simulink model "force_interaction"  (R2016b)
settings: Solver=FixedStepDiscrete  StartTime=0.0  StopTime=10  FixedStep=0.002  RelTol=1e-3
values from neighbouring files (symbols this model uses):
  r_kd = 1.0    [force_interaction.sldd]    (also in init.m = 0)
  r_ki = 1.0    [force_interaction.sldd]    (also in init.m = 0)
  r_kp = 1.0    [force_interaction.sldd]    (also in init.m = 0)
  x_kd = 1.0    [force_interaction.sldd]    (also in init.m = 0)
  x_ki = 1.0    [force_interaction.sldd]    (also in init.m = 0)
  x_kp = 1.0    [force_interaction.sldd]    (also in init.m = 100)
  x_rate = 1000/250    (= 4)    [init.m]
libraries: cstblocks x6, simulink x4
settings Model: Creator=gaoxiao  LastModifiedBy=gx
settings OptimizationCC: DefaultParameterBehavior=Inlined  ZeroExternalMemoryAtStartup=off
settings DebuggingCC: ParameterTunabilityLossMsg=error
settings RTWCC: SystemTargetFile=ert.tlc  GenCodeOnly=on  GenerateMakefile=off  TemplateMakefile=RTW.MSVCBuild  Description=Create Visual C/C++ Solution File for Embedded Coder  GenerateReport=on  IncludeHyperlinkInReport=on  LaunchReport=on  TargetLang=C++  GenerateTraceInfo=on  GenerateTraceReport=on  GenerateTraceReportSl=on  GenerateTraceReportSf=on  GenerateTraceReportEml=on  GenerateWebview=on  GenerateCodeMetricsReport=on
settings CodeAppCC: ForceParamTrailComments=on  OperatorAnnotations=on  SimulinkDataObjDesc=on  SFDataObjDesc=on  MATLABFcnDesc=on  InsertBlockDesc=on  MATLABSourceComments=on
settings ERTTargetCC: TargetLangStandard=C++03 (ISO)  GenerateSampleERTMain=on  MultiInstanceERTCode=on  CodeInterfacePackaging=C++ class  InlinedParameterPlacement=NonHierarchical  RootIOFormat=Structure reference  ERTCustomFileTemplate=example_file_process.tlc  ERTFilePackagingFormat=Compact

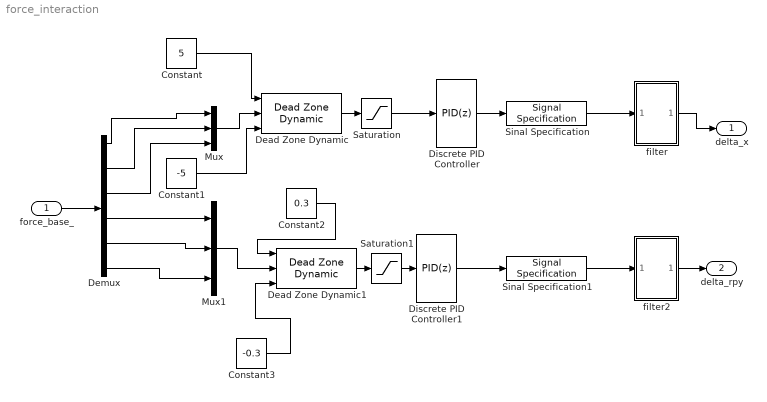
== system force_interaction ==
  force_base_ : Inport  PortDimensions=6
  Constant : Constant  Value=5
  Constant1 : Constant  Value=-5
  Constant2 : Constant  Value=0.3
  Constant3 : Constant  Value=-0.3
  Dead Zone Dynamic : simulink/Discontinuities/Dead Zone Dynamic
  Dead Zone Dynamic1 : simulink/Discontinuities/Dead Zone Dynamic
  Demux : Demux  Outputs=6
  Discrete PID Controller : simulink/Continuous/PID Controller  Controller=PID  TimeDomain=Discrete-time  SampleTime=-1  IntegratorMethod=Forward Euler  FilterMethod=Forward Euler  Form=Parallel  UseFilter=on  ControllerParametersSource=internal  P=x_kp  I=x_ki  D=x_kd  N=5  InitialConditionSource=internal  InitialConditionForIntegrator=0  InitialConditionForFilter=0  ExternalReset=none  LimitOutput=off  UpperSaturationLimit=inf  LowerSaturationLimit=-inf  LinearizeAsGain=off  AntiWindupMode=none  Kb=1  TrackingMode=off  Kt=1  PParamMin=[]  PParamMax=[]  IParamMin=[]  IParamMax=[]  DParamMin=[]  DParamMax=[]  NParamMin=[]  NParamMax=[]  KbParamMin=[]  KbParamMax=[]  KtParamMin=[]  KtParamMax=[]  POutMin=[]  POutMax=[]  IOutMin=[]  IOutMax=[]  DOutMin=[]  DOutMax=[]  NOutMin=[]  NOutMax=[]  KbOutMin=[]  KbOutMax=[]  KtOutMin=[]  KtOutMax=[]  IntegratorOutMin=[]  IntegratorOutMax=[]  FilterOutMin=[]  FilterOutMax=[]  SumOutMin=[]  SumOutMax=[]  SumI1OutMin=[]  SumI1OutMax=[]  SumI2OutMin=[]  SumI2OutMax=[]  SumI3OutMin=[]  SumI3OutMax=[]  SumDOutMin=[]  SumDOutMax=[]  SaturationOutMin=[]  SaturationOutMax=[]  IntegratorContinuousStateAttributes=''  IntegratorStateMustResolveToSignalObject=off  IntegratorRTWStateStorageClass=Auto  FilterContinuousStateAttributes=''  FilterStateMustResolveToSignalObject=off  FilterRTWStateStorageClass=Auto  DifferentiatorICPrevScaledInput=0  DifferentiatorOutMin=[]  DifferentiatorOutMax=[]
  Discrete PID Controller1 : simulink/Continuous/PID Controller  Controller=PID  TimeDomain=Discrete-time  SampleTime=-1  IntegratorMethod=Forward Euler  FilterMethod=Forward Euler  Form=Parallel  UseFilter=on  ControllerParametersSource=internal  P=r_kp  I=r_ki  D=r_kd  N=5  InitialConditionSource=internal  InitialConditionForIntegrator=0  InitialConditionForFilter=0  ExternalReset=none  LimitOutput=off  UpperSaturationLimit=inf  LowerSaturationLimit=-inf  LinearizeAsGain=off  AntiWindupMode=none  Kb=1  TrackingMode=off  Kt=1  PParamMin=[]  PParamMax=[]  IParamMin=[]  IParamMax=[]  DParamMin=[]  DParamMax=[]  NParamMin=[]  NParamMax=[]  KbParamMin=[]  KbParamMax=[]  KtParamMin=[]  KtParamMax=[]  POutMin=[]  POutMax=[]  IOutMin=[]  IOutMax=[]  DOutMin=[]  DOutMax=[]  NOutMin=[]  NOutMax=[]  KbOutMin=[]  KbOutMax=[]  KtOutMin=[]  KtOutMax=[]  IntegratorOutMin=[]  IntegratorOutMax=[]  FilterOutMin=[]  FilterOutMax=[]  SumOutMin=[]  SumOutMax=[]  SumI1OutMin=[]  SumI1OutMax=[]  SumI2OutMin=[]  SumI2OutMax=[]  SumI3OutMin=[]  SumI3OutMax=[]  SumDOutMin=[]  SumDOutMax=[]  SaturationOutMin=[]  SaturationOutMax=[]  IntegratorContinuousStateAttributes=''  IntegratorStateMustResolveToSignalObject=off  IntegratorRTWStateStorageClass=Auto  FilterContinuousStateAttributes=''  FilterStateMustResolveToSignalObject=off  FilterRTWStateStorageClass=Auto  DifferentiatorICPrevScaledInput=0  DifferentiatorOutMin=[]  DifferentiatorOutMax=[]
  Mux : Mux  Inputs=3
  Mux1 : Mux  Inputs=3
  Saturation : Saturate  UpperLimit=40  LowerLimit=-40
  Saturation1 : Saturate  UpperLimit=3  LowerLimit=-3
  Sinal Specification : SignalSpecification  OutDataTypeStr=double  Dimensions=3
  Sinal Specification1 : SignalSpecification  OutDataTypeStr=double  Dimensions=3
  filter : Subsystem
  filter2 : Subsystem
  delta_x : Outport  PortDimensions=3
  delta_rpy : Outport  Port=2  PortDimensions=3
  wires:
  Discrete PID Controller/1 -> Sinal Specification/1
  force_base_/1 -> Demux/1
  Demux/5 -> Mux1/2
  Demux/4 -> Mux1/1
  Demux/6 -> Mux1/3
  Demux/1 -> Mux/1
  Demux/2 -> Mux/2
  Demux/3 -> Mux/3
  Mux/1 -> Dead Zone Dynamic/2
  Discrete PID Controller1/1 -> Sinal Specification1/1
  Mux1/1 -> Dead Zone Dynamic1/2
  Constant/1 -> Dead Zone Dynamic/1
  Constant1/1 -> Dead Zone Dynamic/3
  Constant2/1 -> Dead Zone Dynamic1/1
  Constant3/1 -> Dead Zone Dynamic1/3
  Dead Zone Dynamic/1 -> Saturation/1
  Saturation/1 -> Discrete PID Controller/1
  Dead Zone Dynamic1/1 -> Saturation1/1
  Saturation1/1 -> Discrete PID Controller1/1
  Sinal Specification/1 -> filter/1(In1)
  filter/1(Out1) -> delta_x/1
  Sinal Specification1/1 -> filter2/1(In1)
  filter2/1(Out1) -> delta_rpy/1

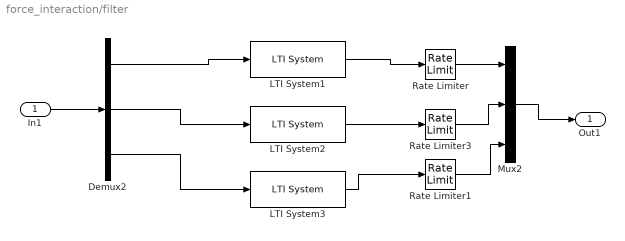
== system force_interaction/filter ==
  In1 : Inport
  Demux2 : Demux  Outputs=3
  LTI System1 : cstblocks/LTI System  sys=TT  IC=[]
  LTI System2 : cstblocks/LTI System  sys=TT  IC=[]
  LTI System3 : cstblocks/LTI System  sys=TT  IC=[]
  Mux2 : Mux  Inputs=3
  Rate Limiter : RateLimiter  RisingSlewLimit=x_rate  FallingSlewLimit=-x_rate  SampleTimeMode=inherited
  Rate Limiter1 : RateLimiter  RisingSlewLimit=x_rate  FallingSlewLimit=-x_rate  SampleTimeMode=inherited
  Rate Limiter3 : RateLimiter  RisingSlewLimit=x_rate  FallingSlewLimit=-x_rate  SampleTimeMode=inherited
  Out1 : Outport
  wires:
  Demux2/2 -> LTI System2/1
  Demux2/1 -> LTI System1/1
  Demux2/3 -> LTI System3/1
  Mux2/1 -> Out1/1
  Rate Limiter3/1 -> Mux2/2
  LTI System3/1 -> Rate Limiter1/1
  Rate Limiter1/1 -> Mux2/3
  Rate Limiter/1 -> Mux2/1
  LTI System2/1 -> Rate Limiter3/1
  LTI System1/1 -> Rate Limiter/1
  In1/1 -> Demux2/1

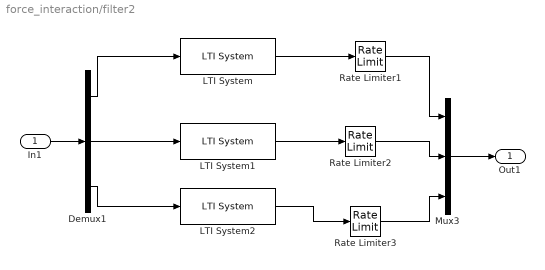
== system force_interaction/filter2 ==
  In1 : Inport
  Demux1 : Demux  Outputs=3
  LTI System : cstblocks/LTI System  sys=TT  IC=[]
  LTI System1 : cstblocks/LTI System  sys=TT  IC=[]
  LTI System2 : cstblocks/LTI System  sys=TT  IC=[]
  Mux3 : Mux  Inputs=3
  Rate Limiter1 : RateLimiter  RisingSlewLimit=x_rate  FallingSlewLimit=-x_rate  SampleTimeMode=inherited
  Rate Limiter2 : RateLimiter  RisingSlewLimit=x_rate  FallingSlewLimit=-x_rate  SampleTimeMode=inherited
  Rate Limiter3 : RateLimiter  RisingSlewLimit=x_rate  FallingSlewLimit=-x_rate  SampleTimeMode=inherited
  Out1 : Outport
  wires:
  LTI System/1 -> Rate Limiter1/1
  LTI System1/1 -> Rate Limiter2/1
  Demux1/2 -> LTI System1/1
  Demux1/1 -> LTI System/1
  Demux1/3 -> LTI System2/1
  Mux3/1 -> Out1/1
  Rate Limiter2/1 -> Mux3/2
  Rate Limiter3/1 -> Mux3/3
  Rate Limiter1/1 -> Mux3/1
  In1/1 -> Demux1/1
  LTI System2/1 -> Rate Limiter3/1
